simulink subsystem "PieroHw"  (R2023b)
settings: Solver=VariableStepAuto  StartTime=0.0  StopTime=10.0  RelTol=1e-3
settings Model: Creator=Hajar  LastModifiedBy=Hajar

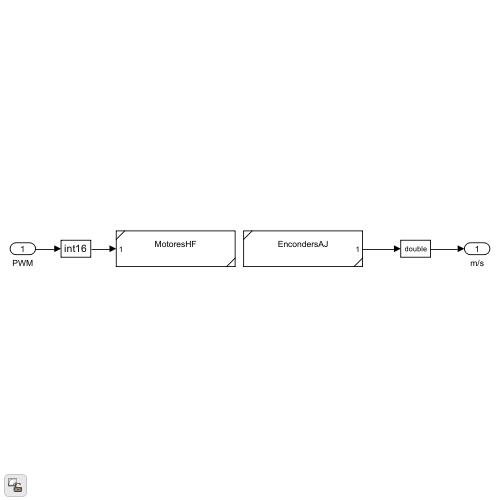
[thumbnail: Simulink's stored preview of the top-level diagram]
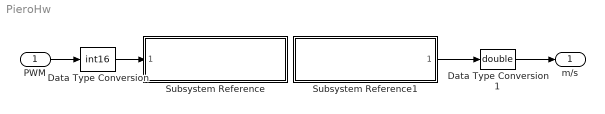
== system PieroHw ==
  PWM : Inport
  Data Type Conversion : DataTypeConversion  OutDataTypeStr=int16  SaturateOnIntegerOverflow=off  RndMeth=Floor
  Data Type Conversion1 : DataTypeConversion  OutDataTypeStr=double  SaturateOnIntegerOverflow=off  RndMeth=Floor
  Subsystem Reference : Subsystem  ReferencedSubsystem=MotoresHF
  Subsystem Reference1 : Subsystem  ReferencedSubsystem=EncondersHF
  m/s : Outport
  wires:
  Subsystem Reference1/1 -> Data Type Conversion1/1
  PWM/1 -> Data Type Conversion/1
  Data Type Conversion1/1 -> m/s/1
  Data Type Conversion/1 -> Subsystem Reference/1
